simulink model "Animation"  (R2017b)
settings: Solver=FixedStepAuto  StartTime=0  StopTime=7  FixedStep=0.01  RelTol=1e-3
values from neighbouring files (symbols this model uses):
  g = 9.81    [specs.mat]
  h = 0.35    [func.m]    (also in specs.mat)
  lf = 1.4    [func.m]    (also in specs.mat)
  lr = 1.345    [func.m]    (also in specs.mat)
  m = 1300    [func.m]    (also in specs.mat)
  r = v/psidot    [func.m]    (also in specs.mat = 0.34)
  wf = 0.85    [func.m]    (also in specs.mat)
  wr = 0.842    [func.m]    (also in specs.mat)
libraries: vrlib x13, sharedtransform x9, simulink x1
settings Model: Creator=Lenovo g505s  LastModifiedBy=Lenovo g505s

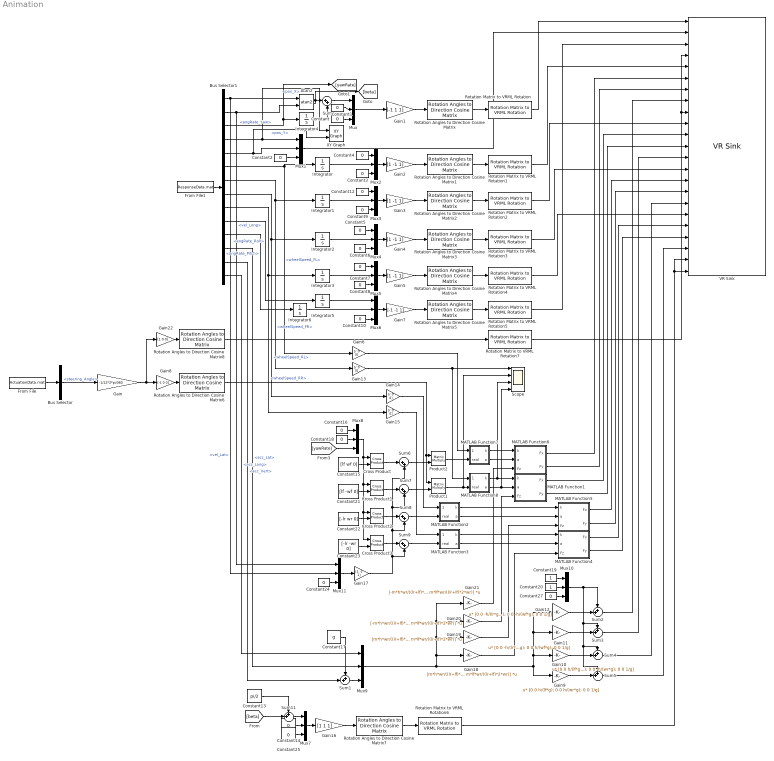
== system Animation ==
  Atan2 : Trigonometry  Operator=atan2
  Bus Selector : BusSelector  OutputSignals=steering_Angle
  Bus Selector1 : BusSelector  OutputSignals=vel_Lat,vel_Long,angRate_Yaw,pos_X,pos_Y,wheelSpeed_FL,wheelSpeed_FR,wheelSpeed_RL,wheelSpeed_RR,angRate_Roll,angRate_Pitch,acc_Lat,acc_Vert,acc_Long
  Constant{,1..10,12,14,16,18,24..25,27} (18 alike) : Constant  Value=0
  Constant13 : Constant  Value=pi/2
  Constant15 : Constant  Value=[lf wf 0]
  Constant17 : Constant  Value=g
  Constant19 : Constant
  Constant20 : Constant
  Constant21 : Constant  Value=[lf -wf 0]
  Constant22 : Constant  Value=[-lr wr 0]
  Constant23 : Constant  Value=[-lr -wr 0]
  Cross Product{,1..3} (4 alike) : vrlib/Utilities/Cross Product
      settings: SourceProductBaseCode=VR
  From File : FromFile  FileName=ActuationData.mat  OutDataTypeStr=Bus: actuation
  From File1 : FromFile  FileName=ResponseData.mat  OutDataTypeStr=Bus: response
  Gain : Gain  Gain=-1/12*2*pi/360
  Gain1 : Gain  Gain=[-1 1 1]
  Gain10 : Gain  Gain=[0 0 h/(lf*g); 0 0 -h/(wr*g); 0 0 1/g]  Multiplication=Matrix(u*K)
  Gain11 : Gain  Gain=[0 0 -h/(lr*g); 0 0 h/(wf*g); 0 0 1/g]  Multiplication=Matrix(u*K)
  Gain12 : Gain  Gain=[0 0 -h/(lr*g); 0 0 -h/(wf*g); 0 0 1/g]  Multiplication=Matrix(u*K)
  Gain{6,13..15} (4 alike) : Gain  Gain=[r 0 0]
  Gain16 : Gain  Gain=[1 1 1]
  Gain{2..5,17} (5 alike) : Gain  Gain=[1 -1 1]
  Gain18 : Gain  Gain=[m*h*wr/((lr+lf)*2*wr) m*h*lf/((lr+lf)*2*wr) m*lf*wr/((lr+lf)*2*wr)]  Multiplication=Matrix(K*u)
  Gain19 : Gain  Gain=[m*h*wr/((lr+lf)*2*wr) -m*h*lf/((lr+lf)*2*wr) m*lf*wr/((lr+lf)*2*wr)]  Multiplication=Matrix(K*u)
  Gain20 : Gain  Gain=[-m*h*wr/((lr+lf)*2*wr) m*h*lf/((lr+lf)*2*wr) m*lf*wr/((lr+lf)*2*wr)]  Multiplication=Matrix(K*u)
  Gain21 : Gain  Gain=[-m*h*wr/((lr+lf)*2*wr) -m*h*lf/((lr+lf)*2*wr) m*lf*wr/((lr+lf)*2*wr)]  Multiplication=Matrix(K*u)
  Gain22 : Gain  Gain=[1 0 0]
  Gain7 : Gain  Gain=[-1 -1 1]
  Gain8 : Gain  Gain=[-1 0 0]
  Gain9 : Gain  Gain=[0 0 h/(lf*g); 0 0 h/(wr*g); 0 0 1/g]  Multiplication=Matrix(u*K)
  Integrator{,1..6} (7 alike) : Integrator
  MATLAB Function1 : MATLAB Function  TreatAsAtomicUnit=on
  MATLAB Function2 : MATLAB Function  TreatAsAtomicUnit=on
  MATLAB Function3 : MATLAB Function  TreatAsAtomicUnit=on
  MATLAB Function4 : MATLAB Function  TreatAsAtomicUnit=on
  MATLAB Function5 : MATLAB Function  TreatAsAtomicUnit=on
  MATLAB Function6 : MATLAB Function  TreatAsAtomicUnit=on
  MATLAB Function7 : MATLAB Function  TreatAsAtomicUnit=on
  MATLAB Function8 : MATLAB Function  TreatAsAtomicUnit=on
  Mux{,1..11} (12 alike) : Mux  Inputs=3
  Product1 : Product  Multiplication=Matrix(*)
  Product2 : Product  Multiplication=Matrix(*)
  Rotation Angles to Direction Cosine Matrix : sharedtransform/Rotation Angles to Direction Cosine Matrix  rotationOrder=ZXY
      settings: SourceProductBaseCode=AE
  Rotation Angles to Direction Cosine Matrix1 : sharedtransform/Rotation Angles to Direction Cosine Matrix  rotationOrder=XYZ
      settings: SourceProductBaseCode=AE
  Rotation Angles to Direction Cosine Matrix2 : sharedtransform/Rotation Angles to Direction Cosine Matrix  rotationOrder=XYZ
      settings: SourceProductBaseCode=AE
  Rotation Angles to Direction Cosine Matrix{3..4,6..8} (5 alike) : sharedtransform/Rotation Angles to Direction Cosine Matrix  rotationOrder=ZYX
      settings: SourceProductBaseCode=AE
  Rotation Angles to Direction Cosine Matrix5 : sharedtransform/Rotation Angles to Direction Cosine Matrix  rotationOrder=XYZ
      settings: SourceProductBaseCode=AE
  Rotation Matrix to VRML Rotation{,1..7} (8 alike) : vrlib/Utilities/Rotation Matrix to VRML Rotation  maxzero=1e-12
      settings: SourceProductName=Simulink 3D Animation  SourceProductBaseCode=VR
  Scope : Scope  NumInputPorts=4
  Sum{,6..9} (5 alike) : Sum  Inputs=|++
  Sum{1..5,11} (6 alike) : Sum  Inputs=++|
  VR Sink : vrlib/VR Sink  InstantiateOnLoad=on  SampleTime=-1  ViewEnable=on  RemoteChange=off  RemoteView=off  FieldsWritten=Car.rotation.4.1.1.double#Car.translation.3.1.1.double#CM.rotation.4.1.1.double#Steering_FL.rotation.4.1.1.double#Wheel_FL_rot.rotation.4.1.1.double#X_axis_FL.scale.3.1.1.double#Y_axis_FL.scale.3.1.1.double#Z_axis_FL.scale.3.1.1.double#Steering_FR.rotation.4.1.1.double#Wheel_FR_rot.rotation.4.1.1.double#X_axis_FR.scale.3.1.1.double#Y_axis_FR.scale.3.1.1.double#Z_axis_FR.scale.3.1.1.double#Wheel_RL_rot.rotation.4.1.1.double#X_axis_RL.scale.3.1.1.double#Y_axis_RL.scale.3.1.1.double#Z_axis_RL.scale.3.1.1.double#Wheel_RR_rot.rotation.4.1.1.double#X_axis_RR.scale.3.1.1.double#Y_axis_RR.scale.3.1.1.double#Z_axis_RR.scale.3.1.1.double#Top_view_camera.orientation.4.1.1.double#Direction.rotation.4.1.1.double  WorldFileName=VRworld.wrl  AutoView=on  VideoDimensions=[]  AllowVariableSize=off
      settings: SourceProductBaseCode=VR
  XY Graph : simulink/Sinks/XY Graph  xmin=-10  xmax=150  ymin=-10  ymax=150  st=-1
  wires:
  From File/1 -> Bus Selector/1
  From File1/1 -> Bus Selector1/1
  Constant1/1 -> Mux/2
  Bus Selector1/4 -> XY Graph/1, Mux1/1  "<pos_X>"
  Rotation Angles to Direction Cosine Matrix/1 -> Rotation Matrix to VRML Rotation/1
  Constant2/1 -> Mux1/3
  Bus Selector1/5 -> XY Graph/2, Mux1/2  "<pos_Y>"
  Bus Selector1/2 -> Atan2/2, Mux11/1  "<vel_Long>"
  Bus Selector1/1 -> Atan2/1, Mux11/2  "<vel_Lat>"
  Mux/1 -> Gain1/1
  Bus Selector/1 -> Gain/1  "<steering_Angle>"
  Bus Selector1/6 -> Integrator/1, Gain6/1  "<wheelSpeed_FL>"
  Bus Selector1/7 -> Gain13/1, Integrator1/1  "<wheelSpeed_FR>"
  Bus Selector1/8 -> Gain14/1, Integrator2/1  "<wheelSpeed_RL>"
  Bus Selector1/9 -> Gain15/1, Integrator3/1  "<wheelSpeed_RR>"
  Rotation Angles to Direction Cosine Matrix3/1 -> Rotation Matrix to VRML Rotation3/1
  Mux4/1 -> Gain4/1
  Integrator2/1 -> Mux4/2
  Constant8/1 -> Mux5/3
  Integrator3/1 -> Mux5/2
  Rotation Angles to Direction Cosine Matrix4/1 -> Rotation Matrix to VRML Rotation4/1
  Constant7/1 -> Mux5/1
  Mux5/1 -> Gain5/1
  Constant/1 -> Mux/3
  Gain1/1 -> Rotation Angles to Direction Cosine Matrix/1
  Gain4/1 -> Rotation Angles to Direction Cosine Matrix3/1
  Gain5/1 -> Rotation Angles to Direction Cosine Matrix4/1
  Bus Selector1/3 -> [yawRate], Integrator4/1  "<angRate_Yaw>"
  Sum/1 -> Mux/1
  Atan2/1 -> [beta], Sum/1
  Integrator4/1 -> Sum/2
  Constant10/1 -> Mux6/3
  Mux6/1 -> Gain7/1
  Rotation Angles to Direction Cosine Matrix5/1 -> Rotation Matrix to VRML Rotation5/1
  Gain7/1 -> Rotation Angles to Direction Cosine Matrix5/1
  Integrator5/1 -> Mux6/1
  Integrator6/1 -> Mux6/2
  Bus Selector1/10 -> Integrator5/1  "<angRate_Roll>"
  Bus Selector1/11 -> Integrator6/1  "<angRate_Pitch>"
  Rotation Angles to Direction Cosine Matrix6/1 -> Product1/1, Product2/1
  Integrator1/1 -> Mux3/2
  Gain3/1 -> Rotation Angles to Direction Cosine Matrix2/1
  Integrator/1 -> Mux2/2
  Mux2/1 -> Gain2/1
  Mux3/1 -> Gain3/1
  Rotation Angles to Direction Cosine Matrix1/1 -> Rotation Matrix to VRML Rotation1/1
  Rotation Angles to Direction Cosine Matrix2/1 -> Rotation Matrix to VRML Rotation2/1
  Gain2/1 -> Rotation Angles to Direction Cosine Matrix1/1
  Bus Selector1/14 -> Mux9/1  "<acc_Long>"
  Bus Selector1/12 -> Mux9/2  "<acc_Lat>"
  Bus Selector1/13 -> Sum1/2  "<acc_Vert>"
  Sum1/1 -> Mux9/3
  Constant17/1 -> Sum1/1
  Constant16/1 -> Mux8/1
  Constant19/1 -> Mux10/1
  Constant20/1 -> Mux10/2
  Constant27/1 -> Mux10/3
  Gain12/1 -> Sum2/2
  Mux10/1 -> Sum4/1, Sum5/1, Sum3/1, Sum2/1
  Gain11/1 -> Sum3/2
  Gain10/1 -> Sum4/2
  Gain9/1 -> Sum5/2
  Constant21/1 -> Cross Product1/2
  Constant22/1 -> Cross Product2/2
  Constant23/1 -> Cross Product3/2
  Mux8/1 -> Cross Product/1, Cross Product2/1, Cross Product3/1, Cross Product1/1
  Constant24/1 -> Mux11/3
  Cross Product2/1 -> Sum8/1
  Cross Product3/1 -> Sum9/1
  Cross Product1/1 -> Sum7/1
  Gain/1 -> Gain22/1, Gain8/1
  Constant5/1 -> Mux4/1
  Gain8/1 -> Rotation Angles to Direction Cosine Matrix6/1
  Constant6/1 -> Mux4/3
  Constant4/1 -> Mux2/1
  Constant12/1 -> Mux3/1
  Gain16/1 -> Rotation Angles to Direction Cosine Matrix7/1
  Mux7/1 -> Gain16/1
  Rotation Angles to Direction Cosine Matrix7/1 -> Rotation Matrix to VRML Rotation6/1
  Constant13/1 -> Sum11/1
  [beta] -> Sum11/2
  Sum11/1 -> Mux7/1
  Constant14/1 -> Mux7/2
  Constant25/1 -> Mux7/3
  Cross Product/1 -> Sum6/1
  Constant15/1 -> Cross Product/2
  Mux11/1 -> Gain17/1
  Constant18/1 -> Mux8/2
  Gain17/1 -> Sum9/2, Sum6/2, Sum7/2, Sum8/2
  [yawRate] -> Mux8/3
  Sum8/1 -> MATLAB Function2/2(real)
  Sum6/1 -> Product2/2
  Gain6/1 -> MATLAB Function7/1(requ)
  Gain14/1 -> MATLAB Function2/1(requ)
  Gain15/1 -> MATLAB Function3/1(requ)
  Sum9/1 -> MATLAB Function3/2(real)
  MATLAB Function3/2(a) -> MATLAB Function4/2(a)
  MATLAB Function3/1(k) -> MATLAB Function4/1(k)
  Mux9/1 -> Gain21/1, Gain20/1, Gain19/1, Gain18/1, Gain9/1, Gain12/1, Gain11/1, Gain10/1
  Gain18/1 -> MATLAB Function4/3(Fz)
  MATLAB Function2/1(k) -> MATLAB Function5/1(k)
  MATLAB Function2/2(a) -> MATLAB Function5/2(a)
  Gain19/1 -> MATLAB Function5/3(Fz)
  MATLAB Function8/1(k) -> MATLAB Function1/1(k), Scope/3
  MATLAB Function8/2(a) -> MATLAB Function1/2(a), Scope/4
  MATLAB Function7/1(k) -> MATLAB Function6/1(k)
  Gain21/1 -> MATLAB Function6/3(Fz)
  Gain20/1 -> MATLAB Function1/3(Fz)
  Product2/1 -> MATLAB Function7/2(real)
  Gain13/1 -> MATLAB Function8/1(requ), Scope/1
  Sum7/1 -> Product1/2
  Product1/1 -> Scope/2, MATLAB Function8/2(real)
  MATLAB Function7/2(a) -> MATLAB Function6/2(a)
  Rotation Matrix to VRML Rotation/1 -> VR Sink/1
  Mux1/1 -> VR Sink/2
  Rotation Matrix to VRML Rotation5/1 -> VR Sink/3
  Rotation Matrix to VRML Rotation1/1 -> VR Sink/5
  MATLAB Function6/1(Fx) -> VR Sink/6
  MATLAB Function6/2(Fy) -> VR Sink/7
  Sum2/1 -> VR Sink/8
  Rotation Matrix to VRML Rotation2/1 -> VR Sink/10
  MATLAB Function1/1(Fx) -> VR Sink/11
  MATLAB Function1/2(Fy) -> VR Sink/12
  Sum3/1 -> VR Sink/13
  Rotation Matrix to VRML Rotation3/1 -> VR Sink/14
  MATLAB Function5/1(Fx) -> VR Sink/15
  MATLAB Function5/2(Fy) -> VR Sink/16
  Sum4/1 -> VR Sink/17
  Rotation Matrix to VRML Rotation4/1 -> VR Sink/18
  MATLAB Function4/1(Fx) -> VR Sink/19
  MATLAB Function4/2(Fy) -> VR Sink/20
  Sum5/1 -> VR Sink/21
  Rotation Matrix to VRML Rotation6/1 -> VR Sink/22, VR Sink/23
  Constant3/1 -> Mux2/3
  Constant9/1 -> Mux3/3
  Rotation Matrix to VRML Rotation7/1 -> VR Sink/4, VR Sink/9
  Gain22/1 -> Rotation Angles to Direction Cosine Matrix8/1
  Rotation Angles to Direction Cosine Matrix8/1 -> Rotation Matrix to VRML Rotation7/1

== matlab function Animation/MATLAB Function1 ==
  data: k input; Fx output; a input; Fz input; Fy output
function [Fx, Fy] = F_x(k, a, Fz)
Fz0 = 3095;
PCX1=1.63;
PDX1=1.06;
PDX2=-0.0492;
PEX1=0.5;
PEX2=-0.11;
PEX3=-0.06;
PEX4=0;
PKX1=19.7;
PKX2=-0.15;
PKX3=0.18;
PHX1=-0.0005;
PHX2=8.5e-5;
PVX1=0;
PVX2=0;
RBX1=9.0;
RBX2=-8.6;
RCX1=1.131;
REX1=0.081;
REX2=-0.15;
RHX1=-0.029;
PCY1=1.28;
PDY1=-0.92;
PDY2=0.22;
PEY1=-1.1;
PEY2=0.65;
PEY3=-0.65;
PKY1=-13.06;
PKY2=1.77;
PHY1=0.0034;
PHY2=-0.003;
PVY1=0.044;
PVY2=-0.030;
RBY1=6.4;
RBY2=7.91;
RBY3=-0.059;
RCY1=1.16;
REY1=0.22;
REY2=0.43;
RHY1=0.0007;
RHY2=0.023;
RVY1=0;
RVY2=0;
RVY4=10;
RVY5=1.94;
RVY6=-50;
 
%k = w*Re/Vx - 1;
dfz = (Fz - Fz0)/Fz0;

Shx = PHX1 + PHX2*dfz;
Svx = Fz * (PVX1 + PVX2 * dfz);
kx = k + Shx;
Cx = PCX1;
Dx = Fz*(PDX1 + PDX2 * dfz);
Ex = (PEX1 + PEX2 * dfz + PEX3 * dfz^2) * (1 - PEX4 * sign(kx));
Bx = Fz * (PKX1 + PKX2 * dfz) * exp(PKX3 * dfz) / (Cx*Dx);
Fx0 = Dx*sin(Cx*atan(Bx*kx - Ex*(Bx*kx - atan(Bx*kx)))) + Svx;

Bxa = RBX1 * cos(atan(RBX2 * k));
Cxa = RCX1;
Exa = REX1 + REX2*dfz;
Shxa = RHX1;
as = a + Shxa;
Gxa = (cos(Cxa*atan(Bxa*as - Exa*(Bxa*as - atan(Bxa*as)))))/...
(cos(Cxa*atan(Bxa*Shxa - Exa*(Bxa*Shxa - atan(Bxa*Shxa)))));

Fx = [(Fx0 * Gxa/Fz0) 1 1];


Shy = PHY1 + PHY2*dfz;
Svy = Fz * (PVY1 + PVY2 * dfz);
ay = a + Shy;
Cy = PCY1;
Dy = Fz*(PDY1 + PDY2 * dfz);
Ey = (PEY1 + PEY2 * dfz) * (1 - PEY3 * sign(ay));
By = PKY1 * Fz0 * sin(2 * atan(Fz/(PKY2 * Fz0)))  / (Cy*Dy);
Fy0 = Dy*sin(Cy*atan(By*ay - Ey*(By*ay - atan(By*ay)))) + Svy;

Svyk = (PDY1 + PDY2*dfz) *Fz*(RVY1 + RVY2*dfz)*...
    cos(atan(RVY4*a))*sin(RVY5 * atan(RVY6*k));
Shyk = RHY1 + RHY2 * dfz;
ks = k + Shyk;
Byk = RBY1 * cos(atan(RBY2 * (a - RBY3)));
Cyk = RCY1;
Eyk = REY1 + REY2*dfz;
Gyk = (cos(Cyk*atan(Byk*ks - Eyk*(Byk*ks - atan(Byk*ks)))))/...
(cos(Cyk*atan(Byk*Shyk - Eyk*(Byk*Shyk - atan(Byk*Shyk)))));

Fy = [1 ((Fy0 * Gyk + Svyk)/Fz0) 1];
end

== matlab function Animation/MATLAB Function6 ==
  data: k input; Fx output; a input; Fz input; Fy output
function [Fx, Fy] = F_x(k, a, Fz)
Fz0 = 3095;
PCX1=1.63;
PDX1=1.06;
PDX2=-0.0492;
PEX1=0.5;
PEX2=-0.11;
PEX3=-0.06;
PEX4=0;
PKX1=19.7;
PKX2=-0.15;
PKX3=0.18;
PHX1=-0.0005;
PHX2=8.5e-5;
PVX1=0;
PVX2=0;
RBX1=9.0;
RBX2=-8.6;
RCX1=1.131;
REX1=0.081;
REX2=-0.15;
RHX1=-0.029;
PCY1=1.28;
PDY1=-0.92;
PDY2=0.22;
PEY1=-1.1;
PEY2=0.65;
PEY3=-0.65;
PKY1=-13.06;
PKY2=1.77;
PHY1=0.0034;
PHY2=-0.003;
PVY1=0.044;
PVY2=-0.030;
RBY1=6.4;
RBY2=7.91;
RBY3=-0.059;
RCY1=1.16;
REY1=0.22;
REY2=0.43;
RHY1=0.0007;
RHY2=0.023;
RVY1=0;
RVY2=0;
RVY4=10;
RVY5=1.94;
RVY6=-50;
 
%k = w*Re/Vx - 1;
dfz = (Fz - Fz0)/Fz0;

Shx = PHX1 + PHX2*dfz;
Svx = Fz * (PVX1 + PVX2 * dfz);
kx = k + Shx;
Cx = PCX1;
Dx = Fz*(PDX1 + PDX2 * dfz);
Ex = (PEX1 + PEX2 * dfz + PEX3 * dfz^2) * (1 - PEX4 * sign(kx));
Bx = Fz * (PKX1 + PKX2 * dfz) * exp(PKX3 * dfz) / (Cx*Dx);
Fx0 = Dx*sin(Cx*atan(Bx*kx - Ex*(Bx*kx - atan(Bx*kx)))) + Svx;

Bxa = RBX1 * cos(atan(RBX2 * k));
Cxa = RCX1;
Exa = REX1 + REX2*dfz;
Shxa = RHX1;
as = a + Shxa;
Gxa = (cos(Cxa*atan(Bxa*as - Exa*(Bxa*as - atan(Bxa*as)))))/...
(cos(Cxa*atan(Bxa*Shxa - Exa*(Bxa*Shxa - atan(Bxa*Shxa)))));

Fx = [(Fx0 * Gxa/Fz0) 1 1];


Shy = PHY1 + PHY2*dfz;
Svy = Fz * (PVY1 + PVY2 * dfz);
ay = a + Shy;
Cy = PCY1;
Dy = Fz*(PDY1 + PDY2 * dfz);
Ey = (PEY1 + PEY2 * dfz) * (1 - PEY3 * sign(ay));
By = PKY1 * Fz0 * sin(2 * atan(Fz/(PKY2 * Fz0)))  / (Cy*Dy);
Fy0 = Dy*sin(Cy*atan(By*ay - Ey*(By*ay - atan(By*ay)))) + Svy;

Svyk = (PDY1 + PDY2*dfz) *Fz*(RVY1 + RVY2*dfz)*...
    cos(atan(RVY4*a))*sin(RVY5 * atan(RVY6*k));
Shyk = RHY1 + RHY2 * dfz;
ks = k + Shyk;
Byk = RBY1 * cos(atan(RBY2 * (a - RBY3)));
Cyk = RCY1;
Eyk = REY1 + REY2*dfz;
Gyk = (cos(Cyk*atan(Byk*ks - Eyk*(Byk*ks - atan(Byk*ks)))))/...
(cos(Cyk*atan(Byk*Shyk - Eyk*(Byk*Shyk - atan(Byk*Shyk)))));

Fy = [1 ((Fy0 * Gyk + Svyk)/Fz0) 1];
end

== matlab function Animation/MATLAB Function2 ==
  data: requ input; k output; real input; a output
function [k, a] = fcn(requ, real)
a = atan2(real(2), real(1));
k = (requ(1) - real(1))/real(1);
end

== matlab function Animation/MATLAB Function3 ==
  data: requ input; k output; real input; a output
function [k, a] = fcn(requ, real)
a = atan2(real(2), real(1));
k = (requ(1) - real(1))/real(1);
end

== matlab function Animation/MATLAB Function4 ==
  data: k input; Fx output; a input; Fz input; Fy output
function [Fx, Fy] = F_x(k, a, Fz)
Fz0 = 3252;
PCX1=1.63;
PDX1=1.06;
PDX2=-0.0492;
PEX1=0.5;
PEX2=-0.11;
PEX3=-0.06;
PEX4=0;
PKX1=19.7;
PKX2=-0.15;
PKX3=0.18;
PHX1=-0.0005;
PHX2=8.5e-5;
PVX1=0;
PVX2=0;
RBX1=9.0;
RBX2=-8.6;
RCX1=1.131;
REX1=0.081;
REX2=-0.15;
RHX1=-0.029;
PCY1=1.28;
PDY1=-0.92;
PDY2=0.22;
PEY1=-1.1;
PEY2=0.65;
PEY3=-0.65;
PKY1=-13.06;
PKY2=1.77;
PHY1=0.0034;
PHY2=-0.003;
PVY1=0.044;
PVY2=-0.030;
RBY1=6.4;
RBY2=7.91;
RBY3=-0.059;
RCY1=1.16;
REY1=0.22;
REY2=0.43;
RHY1=0.0007;
RHY2=0.023;
RVY1=0;
RVY2=0;
RVY4=10;
RVY5=1.94;
RVY6=-50;
 
%k = w*Re/Vx - 1;
dfz = (Fz - Fz0)/Fz0;

Shx = PHX1 + PHX2*dfz;
Svx = Fz * (PVX1 + PVX2 * dfz);
kx = k + Shx;
Cx = PCX1;
Dx = Fz*(PDX1 + PDX2 * dfz);
Ex = (PEX1 + PEX2 * dfz + PEX3 * dfz^2) * (1 - PEX4 * sign(kx));
Bx = Fz * (PKX1 + PKX2 * dfz) * exp(PKX3 * dfz) / (Cx*Dx);
Fx0 = Dx*sin(Cx*atan(Bx*kx - Ex*(Bx*kx - atan(Bx*kx)))) + Svx;

Bxa = RBX1 * cos(atan(RBX2 * k));
Cxa = RCX1;
Exa = REX1 + REX2*dfz;
Shxa = RHX1;
as = a + Shxa;
Gxa = (cos(Cxa*atan(Bxa*as - Exa*(Bxa*as - atan(Bxa*as)))))/...
(cos(Cxa*atan(Bxa*Shxa - Exa*(Bxa*Shxa - atan(Bxa*Shxa)))));

Fx = [(Fx0 * Gxa/Fz) 1 1];


Shy = PHY1 + PHY2*dfz;
Svy = Fz * (PVY1 + PVY2 * dfz);
ay = a + Shy;
Cy = PCY1;
Dy = Fz*(PDY1 + PDY2 * dfz);
Ey = (PEY1 + PEY2 * dfz) * (1 - PEY3 * sign(ay));
By = PKY1 * Fz0 * sin(2 * atan(Fz/(PKY2 * Fz0)))  / (Cy*Dy);
Fy0 = Dy*sin(Cy*atan(By*ay - Ey*(By*ay - atan(By*ay)))) + Svy;

Svyk = (PDY1 + PDY2*dfz) *Fz*(RVY1 + RVY2*dfz)*...
    cos(atan(RVY4*a))*sin(RVY5 * atan(RVY6*k));
Shyk = RHY1 + RHY2 * dfz;
ks = k + Shyk;
Byk = RBY1 * cos(atan(RBY2 * (a - RBY3)));
Cyk = RCY1;
Eyk = REY1 + REY2*dfz;
Gyk = (cos(Cyk*atan(Byk*ks - Eyk*(Byk*ks - atan(Byk*ks)))))/...
(cos(Cyk*atan(Byk*Shyk - Eyk*(Byk*Shyk - atan(Byk*Shyk)))));

Fy = [1 ((Fy0 * Gyk + Svyk)/Fz) 1];
end

== matlab function Animation/MATLAB Function5 ==
  data: k input; Fx output; a input; Fz input; Fy output
function [Fx, Fy] = F_x(k, a, Fz)
Fz0 = 3252;
PCX1=1.63;
PDX1=1.06;
PDX2=-0.0492;
PEX1=0.5;
PEX2=-0.11;
PEX3=-0.06;
PEX4=0;
PKX1=19.7;
PKX2=-0.15;
PKX3=0.18;
PHX1=-0.0005;
PHX2=8.5e-5;
PVX1=0;
PVX2=0;
RBX1=9.0;
RBX2=-8.6;
RCX1=1.131;
REX1=0.081;
REX2=-0.15;
RHX1=-0.029;
PCY1=1.28;
PDY1=-0.92;
PDY2=0.22;
PEY1=-1.1;
PEY2=0.65;
PEY3=-0.65;
PKY1=-13.06;
PKY2=1.77;
PHY1=0.0034;
PHY2=-0.003;
PVY1=0.044;
PVY2=-0.030;
RBY1=6.4;
RBY2=7.91;
RBY3=-0.059;
RCY1=1.16;
REY1=0.22;
REY2=0.43;
RHY1=0.0007;
RHY2=0.023;
RVY1=0;
RVY2=0;
RVY4=10;
RVY5=1.94;
RVY6=-50;
 
%k = w*Re/Vx - 1;
dfz = (Fz - Fz0)/Fz0;

Shx = PHX1 + PHX2*dfz;
Svx = Fz * (PVX1 + PVX2 * dfz);
kx = k + Shx;
Cx = PCX1;
Dx = Fz*(PDX1 + PDX2 * dfz);
Ex = (PEX1 + PEX2 * dfz + PEX3 * dfz^2) * (1 - PEX4 * sign(kx));
Bx = Fz * (PKX1 + PKX2 * dfz) * exp(PKX3 * dfz) / (Cx*Dx);
Fx0 = Dx*sin(Cx*atan(Bx*kx - Ex*(Bx*kx - atan(Bx*kx)))) + Svx;

Bxa = RBX1 * cos(atan(RBX2 * k));
Cxa = RCX1;
Exa = REX1 + REX2*dfz;
Shxa = RHX1;
as = a + Shxa;
Gxa = (cos(Cxa*atan(Bxa*as - Exa*(Bxa*as - atan(Bxa*as)))))/...
(cos(Cxa*atan(Bxa*Shxa - Exa*(Bxa*Shxa - atan(Bxa*Shxa)))));

Fx = [(Fx0 * Gxa/Fz0) 1 1];


Shy = PHY1 + PHY2*dfz;
Svy = Fz * (PVY1 + PVY2 * dfz);
ay = a + Shy;
Cy = PCY1;
Dy = Fz*(PDY1 + PDY2 * dfz);
Ey = (PEY1 + PEY2 * dfz) * (1 - PEY3 * sign(ay));
By = PKY1 * Fz0 * sin(2 * atan(Fz/(PKY2 * Fz0)))  / (Cy*Dy);
Fy0 = Dy*sin(Cy*atan(By*ay - Ey*(By*ay - atan(By*ay)))) + Svy;

Svyk = (PDY1 + PDY2*dfz) *Fz*(RVY1 + RVY2*dfz)*...
    cos(atan(RVY4*a))*sin(RVY5 * atan(RVY6*k));
Shyk = RHY1 + RHY2 * dfz;
ks = k + Shyk;
Byk = RBY1 * cos(atan(RBY2 * (a - RBY3)));
Cyk = RCY1;
Eyk = REY1 + REY2*dfz;
Gyk = (cos(Cyk*atan(Byk*ks - Eyk*(Byk*ks - atan(Byk*ks)))))/...
(cos(Cyk*atan(Byk*Shyk - Eyk*(Byk*Shyk - atan(Byk*Shyk)))));

Fy = [1 ((Fy0 * Gyk + Svyk)/Fz0) 1];
end

== matlab function Animation/MATLAB Function7 ==
  data: requ input; k output; real input; a output
function [k, a] = fcn(requ, real)
a = atan2(real(2), real(1));
k = (requ(1) - real(1))/real(1);
end

== matlab function Animation/MATLAB Function8 ==
  data: requ input; k output; real input; a output
function [k, a] = fcn(requ, real)
a = atan2(real(2), real(1));
k = (requ(1) - real(1))/real(1);
end
